simulink model "esempio1S"  (R2021a)
settings: Solver=VariableStepAuto  StartTime=0.0  StopTime=10.0  RelTol=1e-3
values from neighbouring files (symbols this model uses):
  A = [0 1; 0 -2]    [esempio1.m]    (also in esempio2.m = [-1 -4; 1 -1]; esempio3.m = [-1 -2; 1 -1]; esempio4.m = [0 1; -25 0])
  Ao = A-L*C    [esempio1.m]    (also in esempio2.m; esempio3.m; esempio4.m)
  B = [0; 1]    [esempio1.m]    (also in esempio2.m = [0;1]; esempio3.m = [0;1]; esempio4.m = [0;1])
  Bo = [B L]    [esempio1.m]    (also in esempio2.m; esempio3.m; esempio4.m)
  C = [1 0]    [esempio1.m]    (also in esempio2.m; esempio3.m; esempio4.m = [0 1])
  Co = eye(2)    [esempio1.m]    (also in esempio2.m; esempio3.m; esempio4.m)
  D = 0    [esempio1.m]    (also in esempio2.m; esempio3.m; esempio4.m)
  Do = zeros(2,2)    [esempio1.m]    (also in esempio2.m; esempio3.m; esempio4.m)
settings Model: Creator=itama  LastModifiedBy=itama

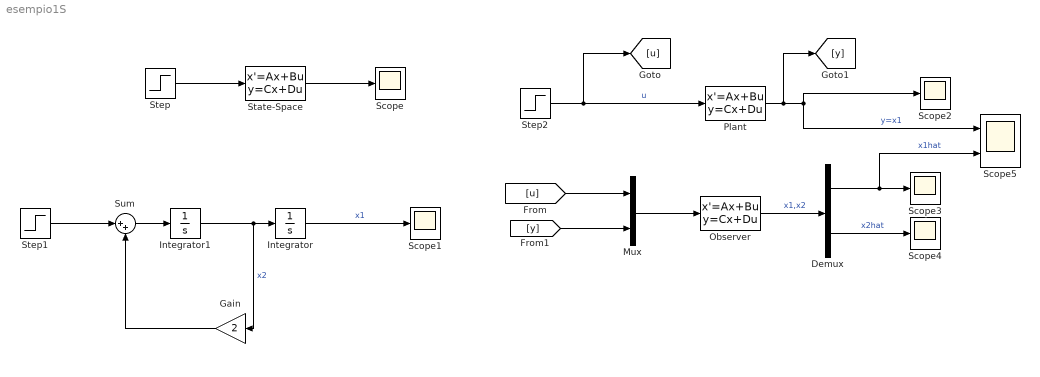
== system esempio1S ==
  Demux : Demux  Outputs=2
  Gain : Gain  Gain=2
  Integrator : Integrator
  Integrator1 : Integrator
  Mux : Mux  Inputs=2
  Observer : StateSpace  A=Ao  B=Bo  C=Co  D=Do  InitialCondition=[0;0]
  Plant : StateSpace  A=A  B=B  C=C  D=D  InitialCondition=[0;0]
  Scope{,1..4} (5 alike) : Scope
  Scope5 : Scope  NumInputPorts=2
  State-Space : StateSpace  A=A  B=B  C=C  D=D  InitialCondition=[0;0]
  Step : Step  SampleTime=0
  Step1 : Step  SampleTime=0
  Step2 : Step  SampleTime=0
  Sum : Sum  Inputs=|++
  wires:
  Step/1 -> State-Space/1
  Integrator/1 -> Scope1/1  "x1"
  State-Space/1 -> Scope/1
  Integrator1/1 -> Gain/1, Integrator/1  "x2"
  Step1/1 -> Sum/1
  Gain/1 -> Sum/2
  Sum/1 -> Integrator1/1
  Step2/1 -> [u], Plant/1  "u"
  Plant/1 -> [y], Scope5/1, Scope2/1  "y=x1"
  Mux/1 -> Observer/1
  Observer/1 -> Demux/1  "x1,x2"
  [u] -> Mux/1
  [y] -> Mux/2
  Demux/1 -> Scope5/2, Scope3/1  "x1hat"
  Demux/2 -> Scope4/1  "x2hat"
